simulink model "DSB_SC_AM_System"  (R2019b)
settings: Solver=VariableStepAuto  StartTime=0.0  StopTime=1  RelTol=1e-3
libraries: simulink x1, dsparch4 x1
settings Model: Creator=SEFA  LastModifiedBy=SEFA

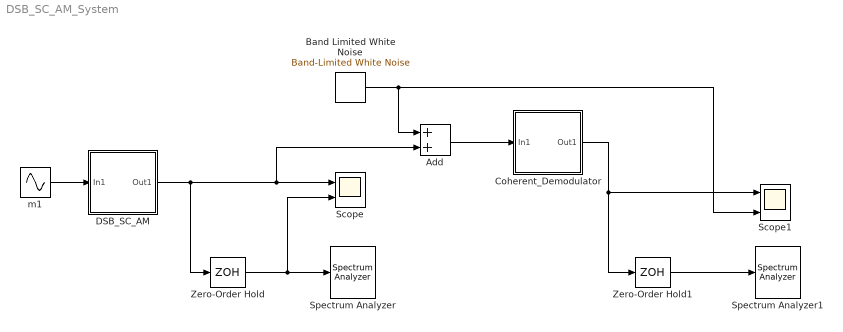
== system DSB_SC_AM_System ==
  Add : Sum
  Band Limited White Noise : simulink/Sources/Band-Limited White Noise  Cov=[0]  Ts=1e-5  seed=[23341]
  Coherent_Demodulator : Subsystem
  DSB_SC_AM : Subsystem
  Scope : Scope  NumInputPorts=2
  Scope1 : Scope  NumInputPorts=2
  Spectrum Analyzer : SpectrumAnalyzer
  Spectrum Analyzer1 : SpectrumAnalyzer
  Zero-Order Hold : ZeroOrderHold  SampleTime=5e-4
  Zero-Order Hold1 : ZeroOrderHold  SampleTime=5e-4
  m1 : Sin  Frequency=2*pi*50  Phase=pi/2  SampleTime=1e-5
  wires:
  DSB_SC_AM/1(Out1) -> Zero-Order Hold/1, Add/2, Scope/1
  m1/1 -> DSB_SC_AM/1(In1)
  Zero-Order Hold/1 -> Scope/2, Spectrum Analyzer/1
  Zero-Order Hold1/1 -> Spectrum Analyzer1/1
  Coherent_Demodulator/1(Out1) -> Zero-Order Hold1/1, Scope1/1
  Add/1 -> Coherent_Demodulator/1(In1)
  Band Limited White Noise/1 -> Add/1, Scope1/2

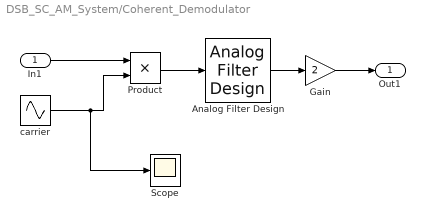
== system DSB_SC_AM_System/Coherent_Demodulator ==
  In1 : Inport
  Analog Filter Design : dsparch4/Analog Filter Design  method=Butterworth  filttype=Lowpass  N=8  Wlo=2*pi*60  Whi=80  Rp=2  Rs=40
  Gain : Gain  Gain=2
  Product : Product
  Scope : Scope
  carrier : Sin  Frequency=2*pi*500  Phase=pi/2  SampleTime=1e-5
  Out1 : Outport
  wires:
  carrier/1 -> Scope/1, Product/2
  In1/1 -> Product/1
  Product/1 -> Analog Filter Design/1
  Analog Filter Design/1 -> Gain/1
  Gain/1 -> Out1/1

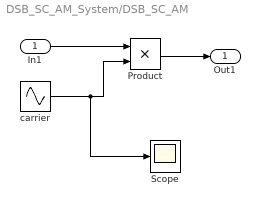
== system DSB_SC_AM_System/DSB_SC_AM ==
  In1 : Inport
  Product : Product
  Scope : Scope
  carrier : Sin  Frequency=2*pi*500  Phase=pi/2  SampleTime=1e-5
  Out1 : Outport
  wires:
  carrier/1 -> Scope/1, Product/2
  In1/1 -> Product/1
  Product/1 -> Out1/1
